simulink model "block_diagram"  (R2017a)
settings: Solver=VariableStepAuto  StartTime=0.0  StopTime=10.0  RelTol=1e-3
settings Model: Creator=Josh  LastModifiedBy=Josh

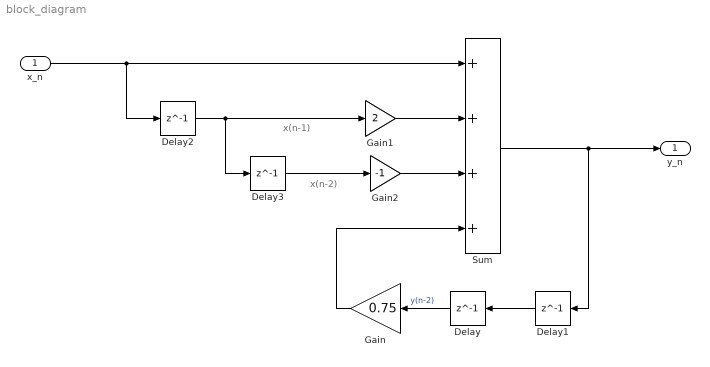
== system block_diagram ==
  note: x(n-2)
  note: x(n-1)
  x_n : Inport
  Delay{,1..3} (4 alike) : Delay  DelayLength=1
  Gain : Gain  Gain=0.75
  Gain1 : Gain  Gain=2
  Gain2 : Gain  Gain=-1
  Sum : Sum  Inputs=++++
  y_n : Outport
  wires:
  Sum/1 -> Delay1/1, y_n/1
  Delay/1 -> Gain/1  "y(n-2)"
  Delay1/1 -> Delay/1
  Gain/1 -> Sum/4
  x_n/1 -> Delay2/1, Sum/1
  Gain1/1 -> Sum/2
  Delay2/1 -> Delay3/1, Gain1/1
  Delay3/1 -> Gain2/1
  Gain2/1 -> Sum/3
